simulink library "quat_degerr_check"  (R2018b)
settings: Solver=VariableStepAuto  StartTime=0.0  StopTime=10.0  RelTol=1e-3
undefined symbols (not defined in the file or in its folder): fsw_params, fswParams
libraries: aerolibutil x2
settings Model: Creator=taylorreynolds  LastModifiedBy=taylorreynolds
settings SFSimCC: SimUseLocalCustomCode=off
settings RTWCC: RTWUseLocalCustomCode=off
settings CodeAppCC: StateflowObjectComments=on

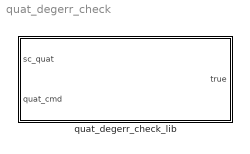
== system quat_degerr_check ==
  quat_degerr_check_lib : Subsystem  mask{point_tol=fsw_params.bus.point_tol}
      mask DialogControl DescTextVar Prompt: Computes the (Euler) angle error between two quaternions and compares to the constant set below. Returns boolean true if the error is less than or equal to the given constant, and false otherwise.

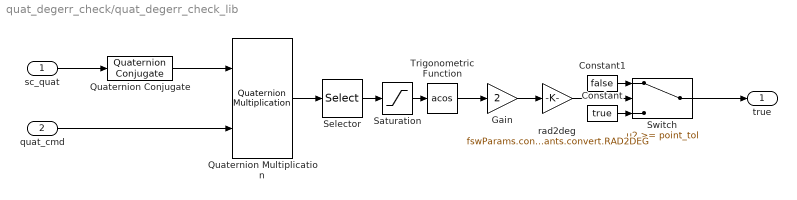
== system quat_degerr_check/quat_degerr_check_lib ==
  sc_quat : Inport
  quat_cmd : Inport  Port=2
  Constant : Constant  Value=true  OutDataTypeStr=boolean
  Constant1 : Constant  Value=false  OutDataTypeStr=boolean
  Gain : Gain  Gain=2
  Quaternion Conjugate : aerolibutil/Quaternion Conjugate
      settings: SourceProductName=Aerospace Blockset  SourceProductBaseCode=AE
  Quaternion Multiplication : aerolibutil/Quaternion Multiplication
  Saturation : Saturate  UpperLimit=1  LowerLimit=-1
  Selector : Selector  InputPortWidth=4  IndexOptions=Index vector (dialog)  Indices=1  OutputSizes=1
  Switch : Switch  Threshold=point_tol
  Trigonometric Function : Trigonometry  Operator=acos
  rad2deg : Gain  Gain=fswParams.constants.convert.RAD2DEG
  true : Outport
  wires:
  Switch/1 -> true/1
  rad2deg/1 -> Switch/2
  Gain/1 -> rad2deg/1
  Trigonometric Function/1 -> Gain/1
  Selector/1 -> Saturation/1
  Quaternion Multiplication/1 -> Selector/1
  quat_cmd/1 -> Quaternion Multiplication/2
  Quaternion Conjugate/1 -> Quaternion Multiplication/1
  sc_quat/1 -> Quaternion Conjugate/1
  Constant/1 -> Switch/3
  Constant1/1 -> Switch/1
  Saturation/1 -> Trigonometric Function/1
